simulink model "pll_final"  (R2013a)
settings: Solver=ode45  StartTime=0.0  StopTime=500*synM/synFr  FixedStep=1/(3*synFr*synN/synM)  MaxStep=.5/(synFr*synN/synM)  RelTol=1e-3
PreLoadFcn:
  | synM = 3;    % frequency division ratio
  | synN = 10;   % frequency division ratio
  | synFr = 30e6;   % reference frequency
  | synFq = synFr;       % quiescent frequency
  | synSen = 40e6;   % VCO sensitivity
libraries: commblksprivate x2, dsparch4 x1, commsynccomp2 x1
CloseFcn:
  | clear synM synN synFr synFq synSen synSigsOut
Description:
  | Phase-Locked Loop (PLL)  Based Frequency Synthesis
  | 
  | This model shows how to simulate a phase-locked loop (PLL) frequency synthesizer.
settings Model: CovMetricSettings=d  ExtModeAutoUpdateStatusClock=off  Creator=The MathWorks Inc.  LastModifiedBy=SALIM AR
settings DataIOCC: SignalLoggingSaveFormat=ModelDataLogs  SaveOutput=off  SaveTime=off  SignalLoggingName=synSigsOut
settings OptimizationCC: BlockReduction=off  BooleanDataType=off  ExpressionDepthLimit=2147483647  InitFltsAndDblsToZero=on  EfficientMapNaN2IntZero=off
settings DebuggingCC: SaveWithParameterizedLinksMsg=none  CheckExecutionContextPreStartOutputMsg=on  CheckExecutionContextRuntimeOutputMsg=on  SignalResolutionControl=TryResolveAllWithWarning  SolverPrmCheckMsg=none  MultiTaskDSMMsg=warning  MultiTaskCondExecSysMsg=none  SigSpecEnsureSampleTimeMsg=none  FcnCallInpInsideContextMsg=UseLocalSettings  StrictBusMsg=None
settings HardwareCC: TargetUnknown=on
settings ModelReferenceCC: UpdateModelReferenceTargets=IfOutOfDate
settings RTWCC: IncludeERTFirstTime=on
settings GRTTargetCC: TargetFcnLib=ansi_tfl_tmw.mat  CombineOutputUpdateFcns=off  GRTInterface=on

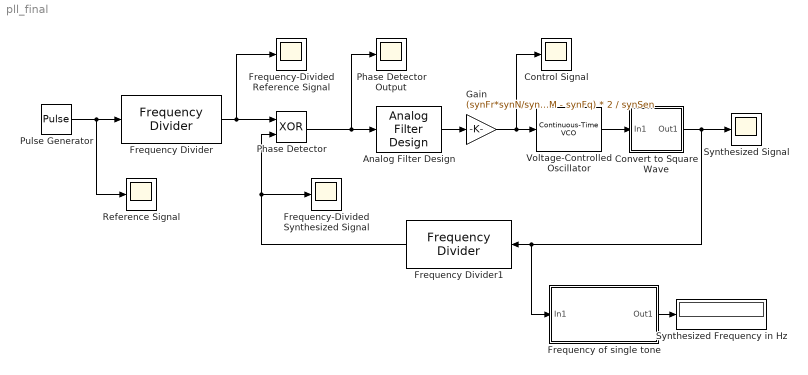
== system pll_final ==
  Analog Filter Design : dsparch4/Analog Filter Design  method=Butterworth  filttype=Lowpass  N=1  Wlo=synFr/synM/10  Whi=80  Rp=2  Rs=40
  Control Signal : Scope
      settings: TimeRange=5e-05  YMin=0  YMax=2.5
  Convert to Square Wave : Subsystem
  Frequency Divider : commblksprivate/Frequency Divider  n=synM
  Frequency Divider1 : commblksprivate/Frequency Divider  n=synN
  Frequency of single tone : Subsystem
      mask Display: disp('Single Tone\nFrequency Estimator');
  Frequency-Divided Reference Signal : Scope
      settings: TimeRange=2e-07  YMin=-1  YMax=2  SaveName=ScopeData5
  Frequency-Divided Synthesized Signal : Scope
      settings: TimeRange=2e-07  YMin=-1  YMax=2  SaveName=ScopeData4
  Gain : Gain  Gain=(synFr*synN/synM - synFq) * 2 / synSen  SaturateOnIntegerOverflow=on  OutDataTypeStr=Inherit: Same as input  ParamDataTypeStr=Inherit: Same as input
  Phase Detector : Logic  Operator=XOR
  Phase Detector Output : Scope
      settings: TimeRange=2e-07  YMin=-1  YMax=2  SaveName=ScopeData6
  Pulse Generator : DiscretePulseGenerator  PulseType=Time based  Period=1/synFr  PulseWidth=50
  Reference Signal : Scope
      settings: TimeRange=1e-07  YMin=-1  YMax=2
  Synthesized Signal : Scope
      settings: TimeRange=5e-08  YMin=-1  YMax=2  SaveName=ScopeData2  MaxDataPoints=50000
  Synthesized Frequency in Hz : Display
  Voltage-Controlled Oscillator : commsynccomp2/Continuous-Time VCO  Ac=1  Fc=synFq  Kc=synSen  Ph=0
  wires:
  Pulse Generator/1 -> Reference Signal/1, Frequency Divider/1
  Phase Detector/1 -> Analog Filter Design/1, Phase Detector Output/1
  Gain/1 -> Voltage-Controlled Oscillator/1, Control Signal/1
  Voltage-Controlled Oscillator/1 -> Convert to Square Wave/1(In1)
  Convert to Square Wave/1(Out1) -> Synthesized Signal/1, Frequency Divider1/1, Frequency of single tone/1(In1)
  Frequency Divider/1 -> Phase Detector/1, Frequency-Divided Reference Signal/1
  Frequency Divider1/1 -> Phase Detector/2, Frequency-Divided Synthesized Signal/1
  Analog Filter Design/1 -> Gain/1
  Frequency of single tone/1(Out1) -> Synthesized Frequency in Hz/1

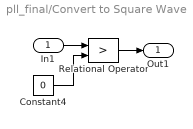
== system pll_final/Convert to Square Wave ==
  In1 : Inport
  Constant4 : Constant  Value=0
  Relational Operator : RelationalOperator  Operator=>  InputSameDT=on
  Out1 : Outport
  wires:
  Relational Operator/1 -> Out1/1
  In1/1 -> Relational Operator/1
  Constant4/1 -> Relational Operator/2

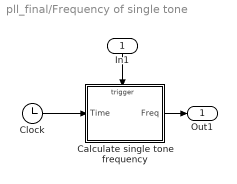
== system pll_final/Frequency of single tone ==
  In1 : Inport
  Calculate single tone frequency : Subsystem  TreatAsAtomicUnit=on
  Clock : Clock
  Out1 : Outport
  wires:
  Calculate single tone frequency/1(Freq) -> Out1/1
  Clock/1 -> Calculate single tone frequency/1(Time)
  In1/1 -> Calculate single tone frequency/Trigger

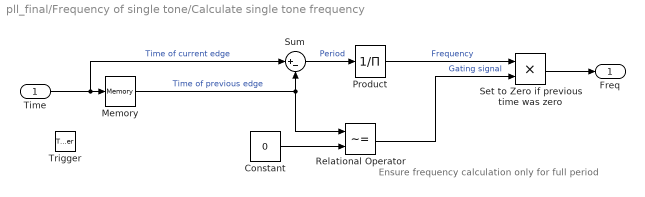
== system pll_final/Frequency of single tone/Calculate single tone frequency ==
  note: Ensure frequency calculation
      | only for full period
  Time : Inport
  Trigger : TriggerPort  ZeroCross=off
  Constant : Constant  Value=0
  Memory : Memory  InheritSampleTime=on
  Product : Product  Inputs=/  SaturateOnIntegerOverflow=on  InputSameDT=on  OutDataTypeStr=Inherit: Same as first input
  Relational Operator : RelationalOperator  Operator=~=  InputSameDT=on
  Set to Zero if previous time was zero : Product  SaturateOnIntegerOverflow=on  InputSameDT=on  OutDataTypeStr=Inherit: Same as first input
  Sum : Sum  Inputs=|+-  SaturateOnIntegerOverflow=on  InputSameDT=on  OutDataTypeStr=Inherit: Same as first input
  Freq : Outport  InitialOutput=0
  wires:
  Relational Operator/1 -> Set to Zero if previous time was zero/2  "Gating signal"
  Constant/1 -> Relational Operator/2
  Set to Zero if previous time was zero/1 -> Freq/1
  Memory/1 -> Relational Operator/1, Sum/2  "Time of previous edge"
  Product/1 -> Set to Zero if previous time was zero/1  "Frequency"
  Sum/1 -> Product/1  "Period"
  Time/1 -> Memory/1, Sum/1  "Time of current edge"
